simulink model "Kinect_Block"  (R2012b)
settings: Solver=ode45  StartTime=0.0  StopTime=inf  RelTol=1e-3
undefined symbols (not defined in the file or in its folder): gray
libraries: nid_lib x2, visionsinks x1, utility x1
settings Model: Creator=Eka  LastModifiedBy=Eka

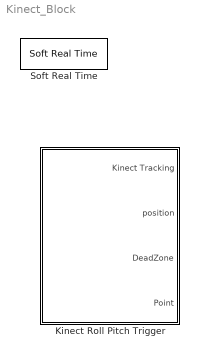
== system Kinect_Block ==
  Kinect Roll Pitch Trigger : Subsystem
  Soft Real Time : utility/Soft Real Time  x=0.8

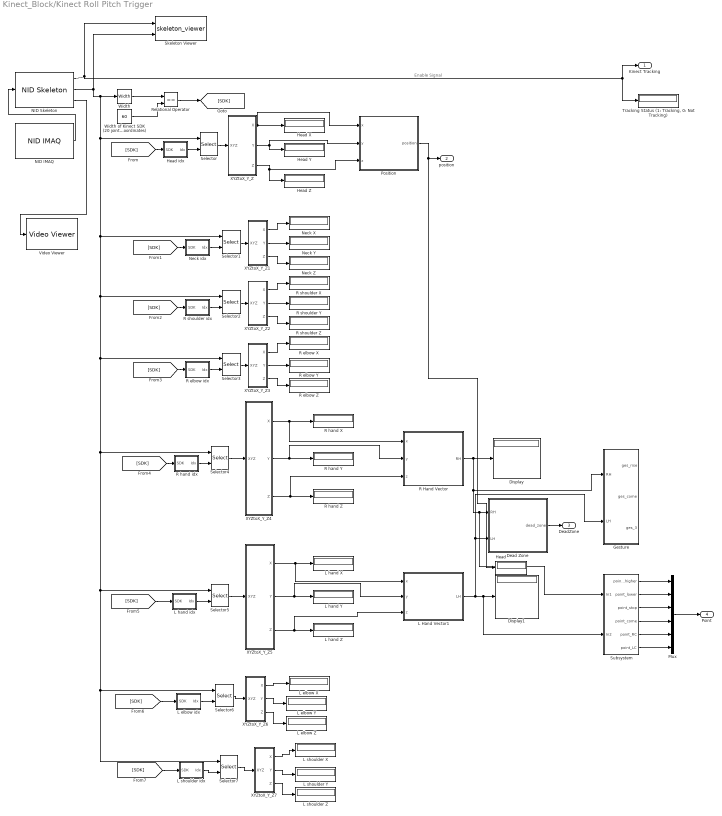
== system Kinect_Block/Kinect Roll Pitch Trigger ==
  note: Enable Signal
  Dead Zone : MATLAB Function  TreatAsAtomicUnit=on
  Display : Display
  Display1 : Display
  Gesture : Subsystem
  Head : Display
  Head X : Display
  Head Y : Display
  Head Z : Display
  Head idx : Subsystem
  L Hand Vector1 : MATLAB Function  TreatAsAtomicUnit=on
  L elbow X : Display
  L elbow Y : Display
  L elbow Z : Display
  L elbow idx : Subsystem
  L hand X : Display
  L hand Y : Display
  L hand Z : Display
  L hand idx : Subsystem
  L shoulder X : Display
  L shoulder Y : Display
  L shoulder Z : Display
  L shoulder idx : Subsystem
  Mux : Mux  Inputs=6
  NID IMAQ : nid_lib/NID IMAQ  imaq_depth=off  imaq_motion=off  imaq_image=off  view_point=off  imaq_skeleton=on  imaq_ir=off  mirror_image=off  imaq_sample_time=1/25  res_fps=VGA (640x480): 30 FPS  needPsiPose=off  angle_input=off  angle=0  angle_read=off  near_mode=on  seated_mode=on  skeleton_smooth=[1.0 0.5 0.5 0.05 0.04]  infer_skeleton=on
  NID Skeleton : nid_lib/NID Skeleton  num_of_skeleton_tracking=1  conv_XYZ_RW=on  viewer=on
  Neck X : Display
  Neck Y : Display
  Neck Z : Display
  Neck idx : Subsystem
  Position : MATLAB Function  TreatAsAtomicUnit=on
  R Hand Vector : MATLAB Function  TreatAsAtomicUnit=on
  R elbow X : Display
  R elbow Y : Display
  R elbow Z : Display
  R elbow idx : Subsystem
  R hand X : Display
  R hand Y : Display
  R hand Z : Display
  R hand idx : Subsystem
  R shoulder X : Display
  R shoulder Y : Display
  R shoulder Z : Display
  R shoulder idx : Subsystem
  Relational Operator : RelationalOperator  Operator===  OutDataTypeStr=boolean
  Selector{,1..7} (8 alike) : Selector  NumberOfDimensions=3  InputPortWidth=3  IndexOptions=Select all,Index vector (port),Select all  Indices=[1 3],1,1  OutputSizes=1,1,1
  Skeleton Viewer : M-S-Function  FunctionName=skeleton_viewer
      mask Display:
      | disp('Skeleton\nViewer')
      | 
      | port_label('input', 1, 'Tracking')
      | port_label('input', 2, 'Skeleton')
  Subsystem : Subsystem
  "Tracking Status (1: Tracking, 0: Not Tracking)" : Display
  Video Viewer : visionsinks/Video Viewer  inputType=Obsolete7b  imagePorts=One multidimensional signal  useColorMap=off  colormapValue=gray(256)  specRange=off  minInputVal=0  maxInputVal=255  FigPos=[691 719 667 610]  AxisZoom=on  trueSizedOnce=off  OpenAtMdlStart=on  DefaultConfigurationName=vipscopes.VideoViewerScopeCfg
  Width : Width
  Width of Kinect SDK (20 joints x 3 coordinates) : Constant  Value=60
  XYZtoX_Y_Z : Subsystem
  XYZtoX_Y_Z1 : Subsystem
  XYZtoX_Y_Z2 : Subsystem
  XYZtoX_Y_Z3 : Subsystem
  XYZtoX_Y_Z4 : Subsystem
  XYZtoX_Y_Z5 : Subsystem
  XYZtoX_Y_Z6 : Subsystem
  XYZtoX_Y_Z7 : Subsystem
  Kinect Tracking : Outport
  position : Outport  Port=2
  DeadZone : Outport  Port=3
  Point : Outport  Port=4
  wires:
  Selector/1 -> XYZtoX_Y_Z/1(XYZ)
  Selector4/1 -> XYZtoX_Y_Z4/1(XYZ)
  Selector3/1 -> XYZtoX_Y_Z3/1(XYZ)
  XYZtoX_Y_Z3/3(Z) -> R elbow Z/1
  XYZtoX_Y_Z3/2(Y) -> R elbow Y/1
  XYZtoX_Y_Z3/1(X) -> R elbow X/1
  Selector2/1 -> XYZtoX_Y_Z2/1(XYZ)
  XYZtoX_Y_Z2/3(Z) -> R shoulder Z/1
  XYZtoX_Y_Z2/2(Y) -> R shoulder Y/1
  XYZtoX_Y_Z2/1(X) -> R shoulder X/1
  XYZtoX_Y_Z1/3(Z) -> Neck Z/1
  XYZtoX_Y_Z1/2(Y) -> Neck Y/1
  XYZtoX_Y_Z1/1(X) -> Neck X/1
  XYZtoX_Y_Z/3(Z) -> Position/3(z), Head Z/1
  [SDK] -> R hand idx/1(SDK)
  R hand idx/1(Idx) -> Selector4/2
  [SDK] -> R elbow idx/1(SDK)
  R elbow idx/1(Idx) -> Selector3/2
  [SDK] -> R shoulder idx/1(SDK)
  R shoulder idx/1(Idx) -> Selector2/2
  Selector1/1 -> XYZtoX_Y_Z1/1(XYZ)
  [SDK] -> Neck idx/1(SDK)
  Neck idx/1(Idx) -> Selector1/2
  XYZtoX_Y_Z/1(X) -> Position/1(x), Head X/1
  NID Skeleton/1 -> "Tracking Status (1: Tracking, 0: Not Tracking)"/1, Kinect Tracking/1, Skeleton Viewer/1
  [SDK] -> Head idx/1(SDK)
  Head idx/1(Idx) -> Selector/2
  Relational Operator/1 -> [SDK]
  Width of Kinect SDK (20 joints x 3 coordinates)/1 -> Relational Operator/2
  Width/1 -> Relational Operator/1
  NID IMAQ/1 -> NID Skeleton/1
  [SDK] -> L hand idx/1(SDK)
  [SDK] -> L elbow idx/1(SDK)
  [SDK] -> L shoulder idx/1(SDK)
  L hand idx/1(Idx) -> Selector5/2
  L elbow idx/1(Idx) -> Selector6/2
  L shoulder idx/1(Idx) -> Selector7/2
  Selector5/1 -> XYZtoX_Y_Z5/1(XYZ)
  XYZtoX_Y_Z6/1(X) -> L elbow X/1
  XYZtoX_Y_Z6/2(Y) -> L elbow Y/1
  XYZtoX_Y_Z6/3(Z) -> L elbow Z/1
  XYZtoX_Y_Z7/1(X) -> L shoulder X/1
  XYZtoX_Y_Z7/2(Y) -> L shoulder Y/1
  XYZtoX_Y_Z7/3(Z) -> L shoulder Z/1
  Selector6/1 -> XYZtoX_Y_Z6/1(XYZ)
  Selector7/1 -> XYZtoX_Y_Z7/1(XYZ)
  NID Skeleton/3 -> Video Viewer/1
  NID Skeleton/2 -> Selector3/1, Selector4/1, Selector6/1, Selector7/1, Selector5/1, Selector2/1, Selector1/1, Selector/1, Width/1, Skeleton Viewer/2
  XYZtoX_Y_Z5/2(Y) -> L Hand Vector1/2(y), L hand Y/1
  XYZtoX_Y_Z5/3(Z) -> L Hand Vector1/3(z), L hand Z/1
  XYZtoX_Y_Z4/1(X) -> R Hand Vector/1(x), R hand X/1
  XYZtoX_Y_Z4/2(Y) -> R Hand Vector/2(y), R hand Y/1
  XYZtoX_Y_Z4/3(Z) -> R Hand Vector/3(z), R hand Z/1
  XYZtoX_Y_Z5/1(X) -> L Hand Vector1/1(x), L hand X/1
  L Hand Vector1/1(LH) -> Gesture/2(LH), Dead Zone/2(LH), Subsystem/2(In2), Display1/1
  R Hand Vector/1(RH) -> Gesture/1(RH), Subsystem/1(In1), Dead Zone/1(RH), Display/1
  XYZtoX_Y_Z/2(Y) -> Position/2(y), Head Y/1
  Position/1(position) -> position/1, Head/1
  Dead Zone/1(dead_zone) -> DeadZone/1
  Subsystem/1(point_higher) -> Mux/1
  Subsystem/5(point_RC) -> Mux/5
  Subsystem/6(point_LC) -> Mux/6
  Subsystem/4(point_come) -> Mux/4
  Subsystem/3(point_stop) -> Mux/3
  Subsystem/2(point_lower) -> Mux/2
  Mux/1 -> Point/1

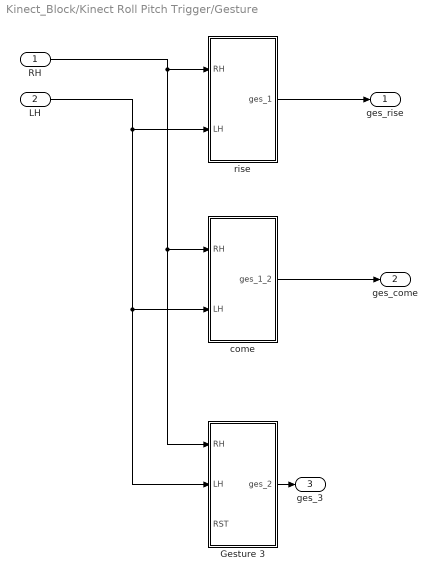
== system Kinect_Block/Kinect Roll Pitch Trigger/Gesture ==
  RH : Inport
  LH : Inport  Port=2
  Gesture 3 : Subsystem
  come : Subsystem
  rise : Subsystem
  ges_rise : Outport
  ges_come : Outport  Port=2
  ges_3 : Outport  Port=3
  wires:
  rise/1(ges_1) -> ges_rise/1
  Gesture 3/1(ges_2) -> ges_3/1
  RH/1 -> Gesture 3/1(RH), come/1(RH), rise/1(RH)
  LH/1 -> come/2(LH), Gesture 3/2(LH), rise/2(LH)
  come/1(ges_1_2) -> ges_come/1

== system Kinect_Block/Kinect Roll Pitch Trigger/Head idx ==
  SDK : Inport
  Kinect SDK : Constant  Value=4
  OpenNI : Constant
  Switch : Switch  Criteria=u2 ~= 0
  Idx : Outport
  wires:
  Switch/1 -> Idx/1
  SDK/1 -> Switch/2
  OpenNI/1 -> Switch/3
  Kinect SDK/1 -> Switch/1

== system Kinect_Block/Kinect Roll Pitch Trigger/L elbow idx ==
  SDK : Inport
  Kinect SDK : Constant  Value=6
  OpenNI : Constant  Value=8
  Switch : Switch  Criteria=u2 ~= 0
  Idx : Outport
  wires:
  Kinect SDK/1 -> Switch/1
  OpenNI/1 -> Switch/3
  SDK/1 -> Switch/2
  Switch/1 -> Idx/1

== system Kinect_Block/Kinect Roll Pitch Trigger/L hand idx ==
  SDK : Inport
  Kinect SDK : Constant  Value=8
  OpenNI : Constant  Value=9
  Switch : Switch  Criteria=u2 ~= 0
  Idx : Outport
  wires:
  Kinect SDK/1 -> Switch/1
  OpenNI/1 -> Switch/3
  SDK/1 -> Switch/2
  Switch/1 -> Idx/1

== system Kinect_Block/Kinect Roll Pitch Trigger/L shoulder idx ==
  SDK : Inport
  Kinect SDK : Constant  Value=5
  OpenNI : Constant  Value=7
  Switch : Switch  Criteria=u2 ~= 0
  Idx : Outport
  wires:
  Kinect SDK/1 -> Switch/1
  OpenNI/1 -> Switch/3
  SDK/1 -> Switch/2
  Switch/1 -> Idx/1

== system Kinect_Block/Kinect Roll Pitch Trigger/Neck idx ==
  SDK : Inport
  Kinect SDK : Constant  Value=3
  OpenNI : Constant  Value=2
  Switch : Switch  Criteria=u2 ~= 0
  Idx : Outport
  wires:
  Kinect SDK/1 -> Switch/1
  OpenNI/1 -> Switch/3
  SDK/1 -> Switch/2
  Switch/1 -> Idx/1

== system Kinect_Block/Kinect Roll Pitch Trigger/R elbow idx ==
  SDK : Inport
  Kinect SDK : Constant  Value=10
  OpenNI : Constant  Value=5
  Switch : Switch  Criteria=u2 ~= 0
  Idx : Outport
  wires:
  Switch/1 -> Idx/1
  SDK/1 -> Switch/2
  OpenNI/1 -> Switch/3
  Kinect SDK/1 -> Switch/1

== system Kinect_Block/Kinect Roll Pitch Trigger/R hand idx ==
  SDK : Inport
  Kinect SDK : Constant  Value=12
  OpenNI : Constant  Value=6
  Switch : Switch  Criteria=u2 ~= 0
  Idx : Outport
  wires:
  Switch/1 -> Idx/1
  SDK/1 -> Switch/2
  OpenNI/1 -> Switch/3
  Kinect SDK/1 -> Switch/1

== system Kinect_Block/Kinect Roll Pitch Trigger/R shoulder idx ==
  SDK : Inport
  Kinect SDK : Constant  Value=9
  OpenNI : Constant  Value=4
  Switch : Switch  Criteria=u2 ~= 0
  Idx : Outport
  wires:
  Switch/1 -> Idx/1
  SDK/1 -> Switch/2
  OpenNI/1 -> Switch/3
  Kinect SDK/1 -> Switch/1

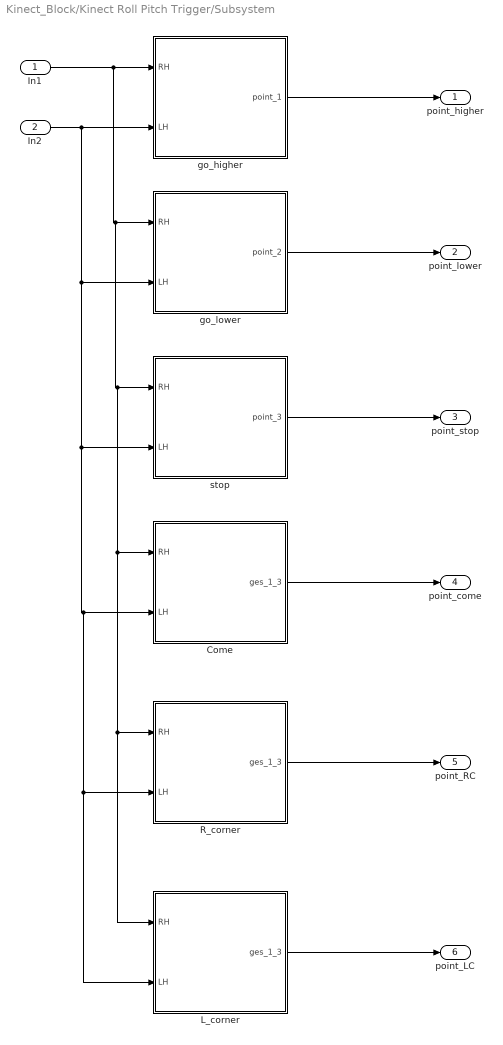
== system Kinect_Block/Kinect Roll Pitch Trigger/Subsystem ==
  In1 : Inport
  In2 : Inport  Port=2
  Come : MATLAB Function  TreatAsAtomicUnit=on
  L_corner : MATLAB Function  TreatAsAtomicUnit=on
  R_corner : MATLAB Function  TreatAsAtomicUnit=on
  go_higher : MATLAB Function  TreatAsAtomicUnit=on
  go_lower : MATLAB Function  TreatAsAtomicUnit=on
  stop : MATLAB Function  TreatAsAtomicUnit=on
  point_higher : Outport
  point_lower : Outport  Port=2
  point_stop : Outport  Port=3
  point_come : Outport  Port=4
  point_RC : Outport  Port=5
  point_LC : Outport  Port=6
  wires:
  go_higher/1(point_1) -> point_higher/1
  stop/1(point_3) -> point_stop/1
  go_lower/1(point_2) -> point_lower/1
  In1/1 -> L_corner/1(RH), R_corner/1(RH), Come/1(RH), stop/1(RH), go_lower/1(RH), go_higher/1(RH)
  In2/1 -> L_corner/2(LH), R_corner/2(LH), Come/2(LH), stop/2(LH), go_lower/2(LH), go_higher/2(LH)
  Come/1(ges_1_3) -> point_come/1
  R_corner/1(ges_1_3) -> point_RC/1
  L_corner/1(ges_1_3) -> point_LC/1

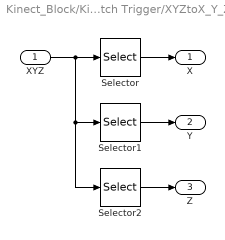
== system Kinect_Block/Kinect Roll Pitch Trigger/XYZtoX_Y_Z ==
  XYZ : Inport
  Selector : Selector  NumberOfDimensions=3  InputPortWidth=3  IndexOptions=Index vector (dialog),Index vector (dialog),Index vector (dialog)  Indices=1,1,1  OutputSizes=1,1,1
  Selector1 : Selector  NumberOfDimensions=3  InputPortWidth=3  IndexOptions=Index vector (dialog),Index vector (dialog),Index vector (dialog)  Indices=1,1,2  OutputSizes=1,1,1
  Selector2 : Selector  NumberOfDimensions=3  InputPortWidth=3  IndexOptions=Index vector (dialog),Index vector (dialog),Index vector (dialog)  Indices=1,1,3  OutputSizes=1,1,1
  X : Outport
  Y : Outport  Port=2
  Z : Outport  Port=3
  wires:
  Selector2/1 -> Z/1
  Selector1/1 -> Y/1
  Selector/1 -> X/1
  XYZ/1 -> Selector2/1, Selector1/1, Selector/1

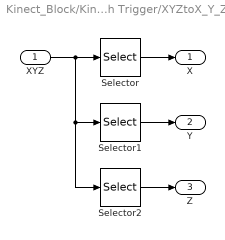
== system Kinect_Block/Kinect Roll Pitch Trigger/XYZtoX_Y_Z1 ==
  XYZ : Inport
  Selector : Selector  NumberOfDimensions=3  InputPortWidth=3  IndexOptions=Index vector (dialog),Index vector (dialog),Index vector (dialog)  Indices=1,1,1  OutputSizes=1,1,1
  Selector1 : Selector  NumberOfDimensions=3  InputPortWidth=3  IndexOptions=Index vector (dialog),Index vector (dialog),Index vector (dialog)  Indices=1,1,2  OutputSizes=1,1,1
  Selector2 : Selector  NumberOfDimensions=3  InputPortWidth=3  IndexOptions=Index vector (dialog),Index vector (dialog),Index vector (dialog)  Indices=1,1,3  OutputSizes=1,1,1
  X : Outport
  Y : Outport  Port=2
  Z : Outport  Port=3
  wires:
  XYZ/1 -> Selector/1, Selector1/1, Selector2/1
  Selector/1 -> X/1
  Selector1/1 -> Y/1
  Selector2/1 -> Z/1

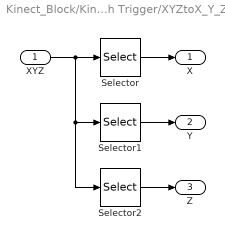
== system Kinect_Block/Kinect Roll Pitch Trigger/XYZtoX_Y_Z2 ==
  XYZ : Inport
  Selector : Selector  NumberOfDimensions=3  InputPortWidth=3  IndexOptions=Index vector (dialog),Index vector (dialog),Index vector (dialog)  Indices=1,1,1  OutputSizes=1,1,1
  Selector1 : Selector  NumberOfDimensions=3  InputPortWidth=3  IndexOptions=Index vector (dialog),Index vector (dialog),Index vector (dialog)  Indices=1,1,2  OutputSizes=1,1,1
  Selector2 : Selector  NumberOfDimensions=3  InputPortWidth=3  IndexOptions=Index vector (dialog),Index vector (dialog),Index vector (dialog)  Indices=1,1,3  OutputSizes=1,1,1
  X : Outport
  Y : Outport  Port=2
  Z : Outport  Port=3
  wires:
  Selector2/1 -> Z/1
  Selector1/1 -> Y/1
  Selector/1 -> X/1
  XYZ/1 -> Selector2/1, Selector1/1, Selector/1

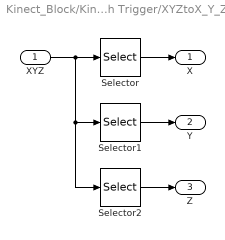
== system Kinect_Block/Kinect Roll Pitch Trigger/XYZtoX_Y_Z3 ==
  XYZ : Inport
  Selector : Selector  NumberOfDimensions=3  InputPortWidth=3  IndexOptions=Index vector (dialog),Index vector (dialog),Index vector (dialog)  Indices=1,1,1  OutputSizes=1,1,1
  Selector1 : Selector  NumberOfDimensions=3  InputPortWidth=3  IndexOptions=Index vector (dialog),Index vector (dialog),Index vector (dialog)  Indices=1,1,2  OutputSizes=1,1,1
  Selector2 : Selector  NumberOfDimensions=3  InputPortWidth=3  IndexOptions=Index vector (dialog),Index vector (dialog),Index vector (dialog)  Indices=1,1,3  OutputSizes=1,1,1
  X : Outport
  Y : Outport  Port=2
  Z : Outport  Port=3
  wires:
  XYZ/1 -> Selector/1, Selector1/1, Selector2/1
  Selector/1 -> X/1
  Selector1/1 -> Y/1
  Selector2/1 -> Z/1

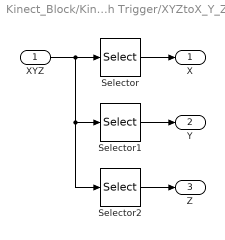
== system Kinect_Block/Kinect Roll Pitch Trigger/XYZtoX_Y_Z4 ==
  XYZ : Inport
  Selector : Selector  NumberOfDimensions=3  InputPortWidth=3  IndexOptions=Index vector (dialog),Index vector (dialog),Index vector (dialog)  Indices=1,1,1  OutputSizes=1,1,1
  Selector1 : Selector  NumberOfDimensions=3  InputPortWidth=3  IndexOptions=Index vector (dialog),Index vector (dialog),Index vector (dialog)  Indices=1,1,2  OutputSizes=1,1,1
  Selector2 : Selector  NumberOfDimensions=3  InputPortWidth=3  IndexOptions=Index vector (dialog),Index vector (dialog),Index vector (dialog)  Indices=1,1,3  OutputSizes=1,1,1
  X : Outport
  Y : Outport  Port=2
  Z : Outport  Port=3
  wires:
  Selector2/1 -> Z/1
  Selector1/1 -> Y/1
  Selector/1 -> X/1
  XYZ/1 -> Selector2/1, Selector1/1, Selector/1

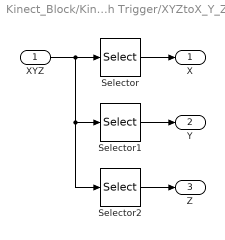
== system Kinect_Block/Kinect Roll Pitch Trigger/XYZtoX_Y_Z5 ==
  XYZ : Inport
  Selector : Selector  NumberOfDimensions=3  InputPortWidth=3  IndexOptions=Index vector (dialog),Index vector (dialog),Index vector (dialog)  Indices=1,1,1  OutputSizes=1,1,1
  Selector1 : Selector  NumberOfDimensions=3  InputPortWidth=3  IndexOptions=Index vector (dialog),Index vector (dialog),Index vector (dialog)  Indices=1,1,2  OutputSizes=1,1,1
  Selector2 : Selector  NumberOfDimensions=3  InputPortWidth=3  IndexOptions=Index vector (dialog),Index vector (dialog),Index vector (dialog)  Indices=1,1,3  OutputSizes=1,1,1
  X : Outport
  Y : Outport  Port=2
  Z : Outport  Port=3
  wires:
  XYZ/1 -> Selector/1, Selector1/1, Selector2/1
  Selector/1 -> X/1
  Selector1/1 -> Y/1
  Selector2/1 -> Z/1

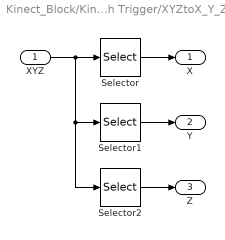
== system Kinect_Block/Kinect Roll Pitch Trigger/XYZtoX_Y_Z6 ==
  XYZ : Inport
  Selector : Selector  NumberOfDimensions=3  InputPortWidth=3  IndexOptions=Index vector (dialog),Index vector (dialog),Index vector (dialog)  Indices=1,1,1  OutputSizes=1,1,1
  Selector1 : Selector  NumberOfDimensions=3  InputPortWidth=3  IndexOptions=Index vector (dialog),Index vector (dialog),Index vector (dialog)  Indices=1,1,2  OutputSizes=1,1,1
  Selector2 : Selector  NumberOfDimensions=3  InputPortWidth=3  IndexOptions=Index vector (dialog),Index vector (dialog),Index vector (dialog)  Indices=1,1,3  OutputSizes=1,1,1
  X : Outport
  Y : Outport  Port=2
  Z : Outport  Port=3
  wires:
  XYZ/1 -> Selector/1, Selector1/1, Selector2/1
  Selector/1 -> X/1
  Selector1/1 -> Y/1
  Selector2/1 -> Z/1

== system Kinect_Block/Kinect Roll Pitch Trigger/XYZtoX_Y_Z7 ==
  XYZ : Inport
  Selector : Selector  NumberOfDimensions=3  InputPortWidth=3  IndexOptions=Index vector (dialog),Index vector (dialog),Index vector (dialog)  Indices=1,1,1  OutputSizes=1,1,1
  Selector1 : Selector  NumberOfDimensions=3  InputPortWidth=3  IndexOptions=Index vector (dialog),Index vector (dialog),Index vector (dialog)  Indices=1,1,2  OutputSizes=1,1,1
  Selector2 : Selector  NumberOfDimensions=3  InputPortWidth=3  IndexOptions=Index vector (dialog),Index vector (dialog),Index vector (dialog)  Indices=1,1,3  OutputSizes=1,1,1
  X : Outport
  Y : Outport  Port=2
  Z : Outport  Port=3
  wires:
  XYZ/1 -> Selector/1, Selector1/1, Selector2/1
  Selector/1 -> X/1
  Selector1/1 -> Y/1
  Selector2/1 -> Z/1

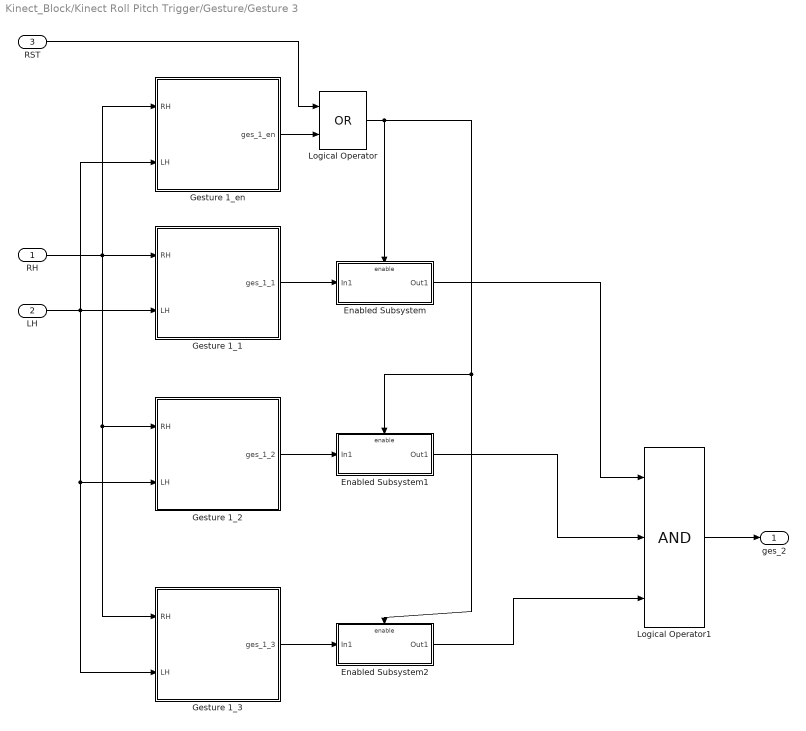
== system Kinect_Block/Kinect Roll Pitch Trigger/Gesture/Gesture 3 ==
  RH : Inport
  LH : Inport  Port=2
  RST : Inport  Port=3
  Enabled Subsystem : Subsystem  TreatAsAtomicUnit=on
  Enabled Subsystem1 : Subsystem  TreatAsAtomicUnit=on
  Enabled Subsystem2 : Subsystem  TreatAsAtomicUnit=on
  Gesture 1_1 : MATLAB Function  TreatAsAtomicUnit=on
  Gesture 1_2 : MATLAB Function  TreatAsAtomicUnit=on
  Gesture 1_3 : MATLAB Function  TreatAsAtomicUnit=on
  Gesture 1_en : MATLAB Function  TreatAsAtomicUnit=on
  Logical Operator : Logic  Operator=OR  AllPortsSameDT=off  OutDataTypeStr=boolean
  Logical Operator1 : Logic  Inputs=3  AllPortsSameDT=off  OutDataTypeStr=boolean
  ges_2 : Outport
  wires:
  RH/1 -> Gesture 1_en/1(RH), Gesture 1_3/1(RH), Gesture 1_2/1(RH), Gesture 1_1/1(RH)
  LH/1 -> Gesture 1_en/2(LH), Gesture 1_3/2(LH), Gesture 1_2/2(LH), Gesture 1_1/2(LH)
  Gesture 1_3/1(ges_1_3) -> Enabled Subsystem2/1(In1)
  Gesture 1_2/1(ges_1_2) -> Enabled Subsystem1/1(In1)
  Gesture 1_1/1(ges_1_1) -> Enabled Subsystem/1(In1)
  Logical Operator/1 -> Enabled Subsystem/Enable, Enabled Subsystem2/Enable, Enabled Subsystem1/Enable
  Gesture 1_en/1(ges_1_en) -> Logical Operator/2
  RST/1 -> Logical Operator/1
  Enabled Subsystem2/1(Out1) -> Logical Operator1/3
  Enabled Subsystem1/1(Out1) -> Logical Operator1/2
  Enabled Subsystem/1(Out1) -> Logical Operator1/1
  Logical Operator1/1 -> ges_2/1

== system Kinect_Block/Kinect Roll Pitch Trigger/Gesture/come ==
  RH : Inport
  LH : Inport  Port=2
  Gesture 1_1 : MATLAB Function  TreatAsAtomicUnit=on
  Gesture 1_2 : MATLAB Function  TreatAsAtomicUnit=on
  Gesture 1_3 : MATLAB Function  TreatAsAtomicUnit=on
  Mux : Mux  Inputs=3
  ges_1_2 : Outport
  wires:
  LH/1 -> Gesture 1_1/2(LH), Gesture 1_2/2(LH), Gesture 1_3/2(LH)
  RH/1 -> Gesture 1_1/1(RH), Gesture 1_3/1(RH), Gesture 1_2/1(RH)
  Mux/1 -> ges_1_2/1
  Gesture 1_1/1(ges_1_1) -> Mux/1
  Gesture 1_2/1(ges_1_2) -> Mux/2
  Gesture 1_3/1(ges_1_3) -> Mux/3

== system Kinect_Block/Kinect Roll Pitch Trigger/Gesture/rise ==
  RH : Inport
  LH : Inport  Port=2
  Gesture 1_1 : MATLAB Function  TreatAsAtomicUnit=on
  Gesture 1_2 : MATLAB Function  TreatAsAtomicUnit=on
  Gesture 1_3 : MATLAB Function  TreatAsAtomicUnit=on
  Mux : Mux  Inputs=3
  ges_1 : Outport
  wires:
  RH/1 -> Gesture 1_3/1(RH), Gesture 1_2/1(RH), Gesture 1_1/1(RH)
  LH/1 -> Gesture 1_3/2(LH), Gesture 1_2/2(LH), Gesture 1_1/2(LH)
  Mux/1 -> ges_1/1
  Gesture 1_1/1(ges_1_1) -> Mux/1
  Gesture 1_2/1(ges_1_2) -> Mux/2
  Gesture 1_3/1(ges_1_3) -> Mux/3

== system Kinect_Block/Kinect Roll Pitch Trigger/Gesture/Gesture 3/Enabled Subsystem ==
  In1 : Inport
  Enable : EnablePort
  Out1 : Outport
  wires:
  In1/1 -> Out1/1

== system Kinect_Block/Kinect Roll Pitch Trigger/Gesture/Gesture 3/Enabled Subsystem1 ==
  In1 : Inport
  Enable : EnablePort
  Out1 : Outport
  wires:
  In1/1 -> Out1/1

== system Kinect_Block/Kinect Roll Pitch Trigger/Gesture/Gesture 3/Enabled Subsystem2 ==
  In1 : Inport
  Enable : EnablePort
  Out1 : Outport
  wires:
  In1/1 -> Out1/1

== matlab function Kinect_Block/Kinect Roll Pitch Trigger/Position ==
  data: x input; y input; z input; position output
function position = fcn(x,y,z)
%#codegen
gx = x*100;
gy = y*100;
gz = z*100;

if (gx > 0 & gx < 10 & ... 
    gy > 70 & gy < 80 & ... 
    gz > 210 & gz < 220)
    
    position = 1;

else
    
    position = 0;

end

== matlab function Kinect_Block/Kinect Roll Pitch Trigger/Dead Zone ==
  data: RH input; LH input; dead_zone output
function dead_zone = fcn(RH, LH)
%#codegen

if (RH(1) > -45 & RH(1) < -16 & ...
    RH(2) > -35 & RH(2) < -20 & ...
    RH(3) > 125 & RH(3) < 165 & ...
    LH(1) > 16 & LH(1) < 45 & ...
    LH(2) > -35 & LH(2) < -20 & ...
    LH(3) > 125 & LH(3) < 165)
    
    dead_zone = 1;

else
    
    dead_zone = 0;

end

== matlab function Kinect_Block/Kinect Roll Pitch Trigger/Gesture/rise/Gesture 1_2 ==
  data: RH input; LH input; ges_1_2 output
function ges_1_2 = fcn(RH, LH)
%#codegen

if (RH(1) > -45 & RH(1) < -30 & ...
    RH(2) > 10 & RH(2) < 30 & ...
    RH(3) > 195 & RH(3) < 220 & ...
    LH(1) > -1000 & LH(1) < 1000 & ...
    LH(2) > -1000 & LH(2) < 1000 & ...
    LH(3) > -1000 & LH(3) < 1000)
    
    ges_1_2 = 1;

else
    
    ges_1_2 = 0;

end

== matlab function Kinect_Block/Kinect Roll Pitch Trigger/L Hand Vector1 ==
  data: x input; y input; z input; LH output
function LH = fcn(x,y,z)
%#codegen
gx = x*100;
gy = y*100;
gz = z*100;
LH = [gx,gy,gz];

== matlab function Kinect_Block/Kinect Roll Pitch Trigger/Gesture/rise/Gesture 1_3 ==
  data: RH input; LH input; ges_1_3 output
function ges_1_3 = fcn(RH, LH)
%#codegen

if (RH(1) > -45 & RH(1) < -30 & ...
    RH(2) > 30 & RH(2) < 50 & ...
    RH(3) > 195 & RH(3) < 220 & ...
    LH(1) > -1000 & LH(1) < 1000 & ...
    LH(2) > -1000 & LH(2) < 1000 & ...
    LH(3) > -1000 & LH(3) < 1000)
    
    ges_1_3 = 1;

else
    
    ges_1_3 = 0;

end

== matlab function Kinect_Block/Kinect Roll Pitch Trigger/Gesture/rise/Gesture 1_1 ==
  data: RH input; LH input; ges_1_1 output
function ges_1_1 = fcn(RH, LH)
%#codegen

if (RH(1) > -45 & RH(1) < -30 & ...
    RH(2) > -10 & RH(2) < 10 & ...
    RH(3) > 195 & RH(3) < 220 & ...
    LH(1) > -1000 & LH(1) < 1000 & ...
    LH(2) > -1000 & LH(2) < 1000 & ...
    LH(3) > -1000 & LH(3) < 1000)
    
    ges_1_1 = 1;

else
    
    ges_1_1 = 0;

end

== matlab function Kinect_Block/Kinect Roll Pitch Trigger/Subsystem/go_higher ==
  data: RH input; LH input; point_1 output
function point_1 = fcn(RH, LH)
%#codegen

if (RH(1) > -55 & RH(1) < -35 & ...
    RH(2) > 45 & RH(2) < 65 & ...
    RH(3) > 200 & RH(3) < 220 & ...
    LH(1) > -1000 & LH(1) < 1000 & ...
    LH(2) > -1000 & LH(2) < 1000 & ...
    LH(3) > -1000 & LH(3) < 1000)
    
    point_1 = 1;

else
    
    point_1 = 0;

end

== matlab function Kinect_Block/Kinect Roll Pitch Trigger/R Hand Vector ==
  data: x input; y input; z input; RH output
function RH = fcn(x,y,z)
%#codegen
gx = x*100;
gy = y*100;
gz = z*100;
RH = [gx,gy,gz];

== matlab function Kinect_Block/Kinect Roll Pitch Trigger/Subsystem/Come ==
  data: RH input; LH input; ges_1_3 output
function ges_1_3 = fcn(RH, LH)
%#codegen

if (RH(1) > -40 & RH(1) < -20 & ...
    RH(2) > 10 & RH(2) < 35 & ...
    RH(3) > 165 & RH(3) < 185 & ...
    LH(1) > -1000 & LH(1) < 1000 & ...
    LH(2) > -1000 & LH(2) < 1000 & ...
    LH(3) > -1000 & LH(3) < 1000)
    
    ges_1_3 = 1;

else
    
    ges_1_3 = 0;

end

== matlab function Kinect_Block/Kinect Roll Pitch Trigger/Gesture/come/Gesture 1_1 ==
  data: RH input; LH input; ges_1_1 output
function ges_1_1 = fcn(RH, LH)
%#codegen

if (RH(1) > -70 & RH(1) < -50 & ...
    RH(2) > 10 & RH(2) < 35 & ...
    RH(3) > 200 & RH(3) < 220 & ...
    LH(1) > -1000 & LH(1) < 1000 & ...
    LH(2) > -1000 & LH(2) < 1000 & ...
    LH(3) > -1000 & LH(3) < 1000)
    
    ges_1_1 = 1;

else
    
    ges_1_1 = 0;

end

== matlab function Kinect_Block/Kinect Roll Pitch Trigger/Gesture/come/Gesture 1_2 ==
  data: RH input; LH input; ges_1_2 output
function ges_1_2 = fcn(RH, LH)
%#codegen

if (RH(1) > -55 & RH(1) < -40 & ...
    RH(2) > 10 & RH(2) < 35 & ...
    RH(3) > 180 & RH(3) < 200 & ...
    LH(1) > -1000 & LH(1) < 1000 & ...
    LH(2) > -1000 & LH(2) < 1000 & ...
    LH(3) > -1000 & LH(3) < 1000)
    
    ges_1_2 = 1;

else
    
    ges_1_2 = 0;

end

== matlab function Kinect_Block/Kinect Roll Pitch Trigger/Gesture/come/Gesture 1_3 ==
  data: RH input; LH input; ges_1_3 output
function ges_1_3 = fcn(RH, LH)
%#codegen

if (RH(1) > -40 & RH(1) < -20 & ...
    RH(2) > 10 & RH(2) < 35 & ...
    RH(3) > 165 & RH(3) < 185 & ...
    LH(1) > -1000 & LH(1) < 1000 & ...
    LH(2) > -1000 & LH(2) < 1000 & ...
    LH(3) > -1000 & LH(3) < 1000)
    
    ges_1_3 = 1;

else
    
    ges_1_3 = 0;

end

== matlab function Kinect_Block/Kinect Roll Pitch Trigger/Subsystem/go_lower ==
  data: RH input; LH input; point_2 output
function point_2 = fcn(RH, LH)
%#codegen

if (RH(1) > -50 & RH(1) < -30 & ...
    RH(2) > -10 & RH(2) < 15 & ...
    RH(3) > 200 & RH(3) < 220 & ...
    LH(1) > -1000 & LH(1) < 1000 & ...
    LH(2) > -1000 & LH(2) < 1000 & ...
    LH(3) > -1000 & LH(3) < 1000)
    
    point_2 = 1;

else
    
    point_2 = 0;

end

== matlab function Kinect_Block/Kinect Roll Pitch Trigger/Subsystem/R_corner ==
  data: RH input; LH input; ges_1_3 output
function ges_1_3 = fcn(RH, LH)
%#codegen

if (RH(1) > -25 & RH(1) < -10 & ...
    RH(2) > 15 & RH(2) < 30 & ...
    RH(3) > 255 & RH(3) < 270 & ...
    LH(1) > -1000 & LH(1) < 1000 & ...
    LH(2) > -1000 & LH(2) < 1000 & ...
    LH(3) > -1000 & LH(3) < 1000)
    
    ges_1_3 = 1;

else
    
    ges_1_3 = 0;

end

== matlab function Kinect_Block/Kinect Roll Pitch Trigger/Gesture/Gesture 3/Gesture 1_1 ==
  data: RH input; LH input; ges_1_1 output
function ges_1_1 = fcn(RH, LH)
%#codegen

if (RH(1) > -50 & RH(1) < -25 & ...
    RH(2) > 10 & RH(2) < 25 & ...
    RH(3) > 130 & RH(3) < 170 & ...
    LH(1) > -1000 & LH(1) < 1000 & ...
    LH(2) > -1000 & LH(2) < 1000 & ...
    LH(3) > -1000 & LH(3) < 1000)
    
    ges_1_1 = 1;

else
    
    ges_1_1 = 0;

end

== matlab function Kinect_Block/Kinect Roll Pitch Trigger/Gesture/Gesture 3/Gesture 1_2 ==
  data: RH input; LH input; ges_1_2 output
function ges_1_2 = fcn(RH, LH)
%#codegen

if (RH(1) > -50 & RH(1) < -25 & ...
    RH(2) > 25 & RH(2) < 40 & ...
    RH(3) > 130 & RH(3) < 170 & ...
    LH(1) > -1000 & LH(1) < 1000 & ...
    LH(2) > -1000 & LH(2) < 1000 & ...
    LH(3) > -1000 & LH(3) < 1000)
    
    ges_1_2 = 1;

else
    
    ges_1_2 = 0;

end

== matlab function Kinect_Block/Kinect Roll Pitch Trigger/Gesture/Gesture 3/Gesture 1_3 ==
  data: RH input; LH input; ges_1_3 output
function ges_1_3 = fcn(RH, LH)
%#codegen

if (RH(1) > -50 & RH(1) < -25 & ...
    RH(2) > 40 & RH(2) < 55 & ...
    RH(3) > 130 & RH(3) < 170 & ...
    LH(1) > -1000 & LH(1) < 1000 & ...
    LH(2) > -1000 & LH(2) < 1000 & ...
    LH(3) > -1000 & LH(3) < 1000)
    
    ges_1_3 = 1;

else
    
    ges_1_3 = 0;

end

== matlab function Kinect_Block/Kinect Roll Pitch Trigger/Subsystem/stop ==
  data: RH input; LH input; point_3 output
function point_3 = fcn(RH, LH)
%#codegen

if (RH(1) > -40 & RH(1) < -20 & ...
    RH(2) > 75 & RH(2) < 90 & ...
    RH(3) > 200 & RH(3) < 235 & ...
    LH(1) > -1000 & LH(1) < 1000 & ...
    LH(2) > -1000 & LH(2) < 1000 & ...
    LH(3) > -1000 & LH(3) < 1000)
    
    point_3 = 1;

else
    
    point_3 = 0;

end

== matlab function Kinect_Block/Kinect Roll Pitch Trigger/Gesture/Gesture 3/Gesture 1_en ==
  data: RH input; LH input; ges_1_en output
function ges_1_en = fcn(RH, LH)
%#codegen

if (RH(1) > -50 & RH(1) < -25 & ...
    RH(2) > 10 & RH(2) < 55 & ...
    RH(3) > 130 & RH(3) < 170 & ...
    LH(1) > -1000 & LH(1) < 1000 & ...
    LH(2) > -1000 & LH(2) < 1000 & ...
    LH(3) > -1000 & LH(3) < 1000)
    
    ges_1_en = 1;

else
    
    ges_1_en = 0;

end

== matlab function Kinect_Block/Kinect Roll Pitch Trigger/Subsystem/L_corner ==
  data: RH input; LH input; ges_1_3 output
function ges_1_3 = fcn(RH, LH)
%#codegen

if (RH(1) > -1000 & RH(1) < 1000 & ...
    RH(2) > -1000 & RH(2) < 1000 & ...
    RH(3) > -1000 & RH(3) < 1000 & ...
    LH(1) > 35 & LH(1) < 55 & ...
    LH(2) > 25 & LH(2) < 45 & ...
    LH(3) > 255 & LH(3) < 270)
    
    ges_1_3 = 1;

else
    
    ges_1_3 = 0;

end
